simulink model "MSFartoystyring"  (R2015b)
settings: Solver=ode45  StartTime=tstart  StopTime=tstop  RelTol=1e-3
values from neighbouring files (symbols this model uses):
  c = 0    [matlab.mat]    (also in run.m; run_2_3.m = 1; test.m)
  psi0 = 0    [matlab.mat]    (also in run.m; run_2_3.m; test.m)
  r0 = 0    [matlab.mat]    (also in run.m; run_2_3.m; test.m)
  tsamp = 10    [matlab.mat]    (also in run.m; run_2_3.m; test.m)
  v0 = [6.63 0]    [matlab.mat]    (also in run.m = [6.63 0]'; run_2_3.m = [6.63 0]'; test.m = [6.63 0]')
undefined symbols (not defined in the file or in its folder): delta_c, delta_offset, msfartoystyring
undefined symbols (not defined in the file): p0
settings Model: ExtModeAutoUpdateStatusClock=off  Creator=christh  LastModifiedBy=ShivJeet
settings DataIOCC: SaveFormat=Array  SignalLoggingSaveFormat=ModelDataLogs
settings OptimizationCC: ExpressionDepthLimit=2147483647  InitFltsAndDblsToZero=on
settings DebuggingCC: UnderspecifiedInitializationDetection=Classic  MergeDetectMultiDrivingBlocksExec=none  SolverPrmCheckMsg=warning  FcnCallInpInsideContextMsg=UseLocalSettings  StateNameClashWarn=warning
settings HardwareCC: ProdBitPerPointer=32  ProdLargestAtomicFloat=None  ProdIntDivRoundTo=Undefined  ProdEndianess=Unspecified  ProdWordSize=32  ProdHWDeviceType=32-bit Generic
settings GRTTargetCC: GeneratePreprocessorConditionals=Disable all  CombineOutputUpdateFcns=off  GRTInterface=on
settings ConfigComp: CovModelRefEnable=Off

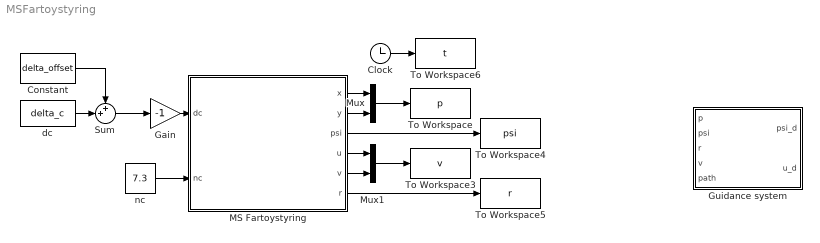
== system MSFartoystyring ==
  Clock : Clock
  Constant : Constant  Value=delta_offset
  Gain : Gain  Gain=-1
  Guidance system : Subsystem
  MS Fartoystyring : Subsystem  mask(MS Fartoystyring for Assignment 3 G&C){x0=p0(1), y0=p0(2), u0=v0(1), v0=v0(2), psi0=psi0, r0=r0, c=c}
      mask prompts: x0 "x(t0) (m)"; y0 "y(t0) (m)"; u0 "u(t0) (m/s)"; v0 "v(t0) (m/s)"; psi0 "psi(t0) (rad)"; r0 "r(t0) (rad/s)"; c "current (0 or 1)"
      mask help:
      | Block corresponding to Figure 1 in the assignment text. Gives the response of the ship.
      |
      | The design speed of MS Fartoystyring is u=8.23 m/s.
      |
      | Input:
      | dc: commanded rudder (rad), dmax=25*pi/180
      | nc: commanded shaft speed (rad/s), nmax=85*2*pi/60
      |
      | Output:
      | x: north pos (m)
      | y: east pos (m)
      | u: surge (m/s)
      | v: sway (m/s)
      | psi: heading (rad)
      | r: yaw (rad/s)
      mask Help: Comments, bugs and help requests can be directed to the TA. Email on course website.
  Mux : Mux  Inputs=2
  Mux1 : Mux  Inputs=2
  Sum : Sum  Inputs=++|
  To Workspace : ToWorkspace  VariableName=p  SampleTime=tsamp
  To Workspace3 : ToWorkspace  VariableName=v  SampleTime=tsamp
  To Workspace4 : ToWorkspace  VariableName=psi  SampleTime=tsamp
  To Workspace5 : ToWorkspace  VariableName=r  SampleTime=tsamp
  To Workspace6 : ToWorkspace  VariableName=t  SampleTime=tsamp
  dc : Constant  Value=delta_c
  nc : Constant  Value=7.3
  wires:
  Clock/1 -> To Workspace6/1
  MS Fartoystyring/1(x) -> Mux/1
  MS Fartoystyring/2(y) -> Mux/2
  MS Fartoystyring/4(u) -> Mux1/1
  MS Fartoystyring/5(v) -> Mux1/2
  Mux/1 -> To Workspace/1
  Mux1/1 -> To Workspace3/1
  MS Fartoystyring/3(psi) -> To Workspace4/1
  MS Fartoystyring/6(r) -> To Workspace5/1
  nc/1 -> MS Fartoystyring/2(nc)
  Gain/1 -> MS Fartoystyring/1(dc)
  dc/1 -> Sum/2
  Sum/1 -> Gain/1
  Constant/1 -> Sum/1

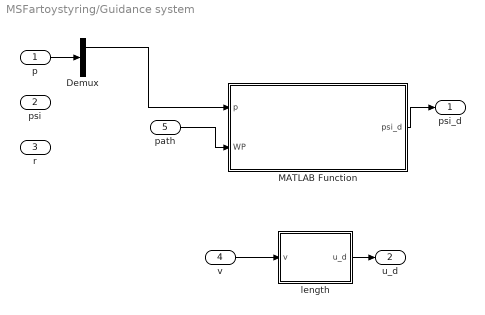
== system MSFartoystyring/Guidance system ==
  p : Inport
  psi : Inport  Port=2
  r : Inport  Port=3
  v : Inport  Port=4
  path : Inport  Port=5
  Demux : Demux  Outputs=2
  MATLAB Function : MATLAB Function  TreatAsAtomicUnit=on
  length : MATLAB Function  TreatAsAtomicUnit=on
  psi_d : Outport
  u_d : Outport  Port=2
  wires:
  p/1 -> Demux/1
  Demux/1 -> MATLAB Function/1(p)
  v/1 -> length/1(v)
  length/1(u_d) -> u_d/1
  ? -> ?
  path/1 -> MATLAB Function/2(WP)
  MATLAB Function/1(psi_d) -> psi_d/1

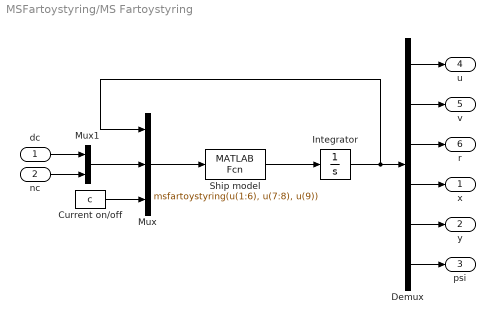
== system MSFartoystyring/MS Fartoystyring ==
  dc : Inport
  nc : Inport  Port=2
  Current on/off : Constant  Value=c
  Demux : Demux  Outputs=6
  Integrator : Integrator  InitialCondition=[u0 v0 r0 x0 y0 psi0]'
  Mux : Mux  Inputs=3
  Mux1 : Mux  Inputs=2
  Ship model : MATLABFcn  MATLABFcn=msfartoystyring(u(1:6), u(7:8), u(9))  OutputDimensions=6
  x : Outport
  y : Outport  Port=2
  psi : Outport  Port=3
  u : Outport  Port=4
  v : Outport  Port=5
  r : Outport  Port=6
  wires:
  Integrator/1 -> Mux/1, Demux/1
  Mux1/1 -> Mux/2
  dc/1 -> Mux1/1
  nc/1 -> Mux1/2
  Demux/1 -> u/1
  Demux/2 -> v/1
  Demux/3 -> r/1
  Demux/4 -> x/1
  Demux/5 -> y/1
  Demux/6 -> psi/1
  Current on/off/1 -> Mux/3
  Ship model/1 -> Integrator/1
  Mux/1 -> Ship model/1

== matlab function MSFartoystyring/Guidance system/length ==
  data: v input; u_d output
function u_d = fcn(v)
%#codegen
u_d = sqrt(v(1)^2 +v(2)^2);
end

== matlab function MSFartoystyring/Guidance system/MATLAB Function ==
  data: p input; psi_d output; WP input
function psi_d  = fcn(p,WP)
persistent index

% Setting the index first time
if isempty(index)
    index = 1;
end

% Waypoint reached, moving to next waypoint
if(p(1) == WP(1,index) && p(2) == WP(2,index))
    index = index + 1;
end

psi_d = atan2(WP(1,index)-p(1),WP(2,index)-p(2));
end
